simulink model "pundul2_sim"  (R2015a)
settings: Solver=ode45  StartTime=0.0  StopTime=15  RelTol=1e-3
values from neighbouring files (symbols this model uses):
  filter_den = [filter_tau 1]    [pendul2.m]
  filter_num = [filter_gain]    [pendul2.m]
  motor_den = [Rm/Lm 1]    [pendul.m]    (also in pendul2.m = [motor_tau 1])
  motor_num = [Rm/Lm]    [pendul.m]    (also in pendul2.m = [motor_tau 0])
  pendul_den = [l 0 -g]    [pendul2.m]
  pendul_num = [1]    [pendul2.m]
  regulator_den = Gc_den{1,1}    [pendul2.m]
  regulator_num = Gc_num{1,1}    [pendul2.m]
undefined symbols (not defined in the file or in its folder): bil_den, bil_num
libraries: dspsrcs4 x1
settings Model: Creator=jorn  LastModifiedBy=jorn

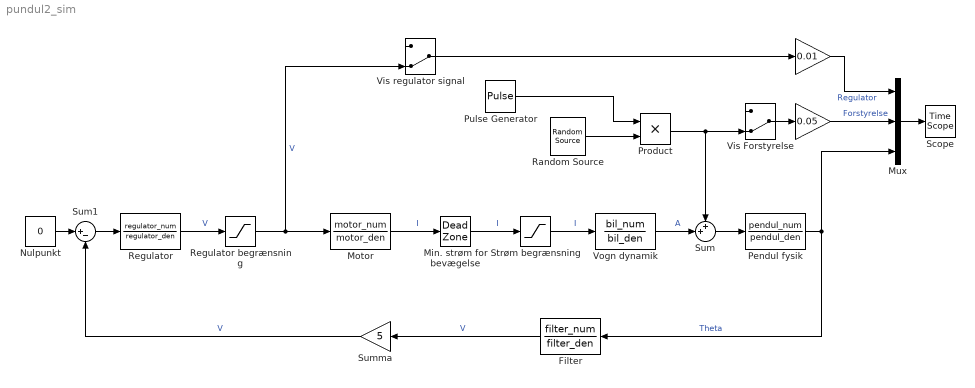
== system pundul2_sim ==
  " " : Gain  Gain=0.05
  "  " : Gain  Gain=0.01
  "Filter " : TransferFcn  Numerator=filter_num  Denominator=filter_den
  Min. strøm for bevægelse : DeadZone  LowerValue=-1  UpperValue=1  SaturateOnIntegerOverflow=on
  Motor : TransferFcn  Numerator=motor_num  Denominator=motor_den
  Mux : Mux  Inputs=3
  Nulpunkt : Constant  Value=0
  Pendul fysik : TransferFcn  Numerator=pendul_num  Denominator=pendul_den
  Product : Product
  Pulse Generator : DiscretePulseGenerator  PulseType=Time based  PulseWidth=5
  Random Source : dspsrcs4/Random Source  SrcType=Uniform  NormMethod=Ziggurat  CltLength=12  MinVal=-1  MaxVal=1  MeanVal=0  VarVal=1  RepMode=Not repeatable  rawSeed=1  IsInherit=off  SampMode=Discrete  SampTime=1  SampFrame=1  DataType=Double  OutComplex=Real
  Regulator : TransferFcn  Numerator=regulator_num  Denominator=regulator_den
  Regulator begrænsning : Saturate  UpperLimit=6  LowerLimit=-6
  Scope : TimeScope
  Strøm begrænsning : Saturate  UpperLimit=1.5  LowerLimit=-1.5
  Sum : Sum  Inputs=++|
  Sum1 : Sum  Inputs=|+-
  Summa : Gain  Gain=5
  Vis Forstyrelse : ManualSwitch  CurrentSetting=0
  Vis regulator signal : ManualSwitch  CurrentSetting=0
  Vogn dynamik : TransferFcn  Numerator=bil_num  Denominator=bil_den
  wires:
  Pendul fysik/1 -> Mux/3, "Filter "/1  "Theta"
  Vogn dynamik/1 -> Sum/2  "A"
  Sum/1 -> Pendul fysik/1
  "Filter "/1 -> Summa/1  "V"
  Nulpunkt/1 -> Sum1/1
  Mux/1 -> Scope/1
  Summa/1 -> Sum1/2  "V"
  Min. strøm for bevægelse/1 -> Strøm begrænsning/1  "I"
  Strøm begrænsning/1 -> Vogn dynamik/1  "I"
  Motor/1 -> Min. strøm for bevægelse/1  "I"
  Regulator/1 -> Regulator begrænsning/1  "V"
  Sum1/1 -> Regulator/1
  Regulator begrænsning/1 -> Motor/1, Vis regulator signal/2  "V"
  " "/1 -> Mux/2  "Forstyrelse"
  Vis Forstyrelse/1 -> " "/1
  Pulse Generator/1 -> Product/1
  Random Source/1 -> Product/2
  Product/1 -> Sum/1, Vis Forstyrelse/2
  Vis regulator signal/1 -> "  "/1
  "  "/1 -> Mux/1  "Regulator"
